simulink model "Batteriemodelle_vergleich"  (R2020a)
settings: Solver=ode15s  StartTime=0.0  StopTime=10.0  MaxStep=1  RelTol=1e-3  AbsTol=1e-3
undefined symbols (not defined in the file or in its folder): c_Mo, J_T, L, M_l, R_a, R_i, R_v, switch_12, switch_48, switch_gen, U_b0
libraries: fl_lib x20, nesl_utility x11, ee_lib x1
settings Model: Creator=ferdi  LastModifiedBy=ferdi
settings SolverCC: AutoScaleAbsTol=off
settings DebuggingCC: SymbolicDimsDataTypeCodeGenerationDiagnostic=none
settings SFSimCC: CustomCodeUndefinedFunction=UseInterfaceOnly
settings SimscapeCC: SimscapeLogType=all  SimscapeLogSimulationStatistics=on  SimscapeLogDataHistory=10000

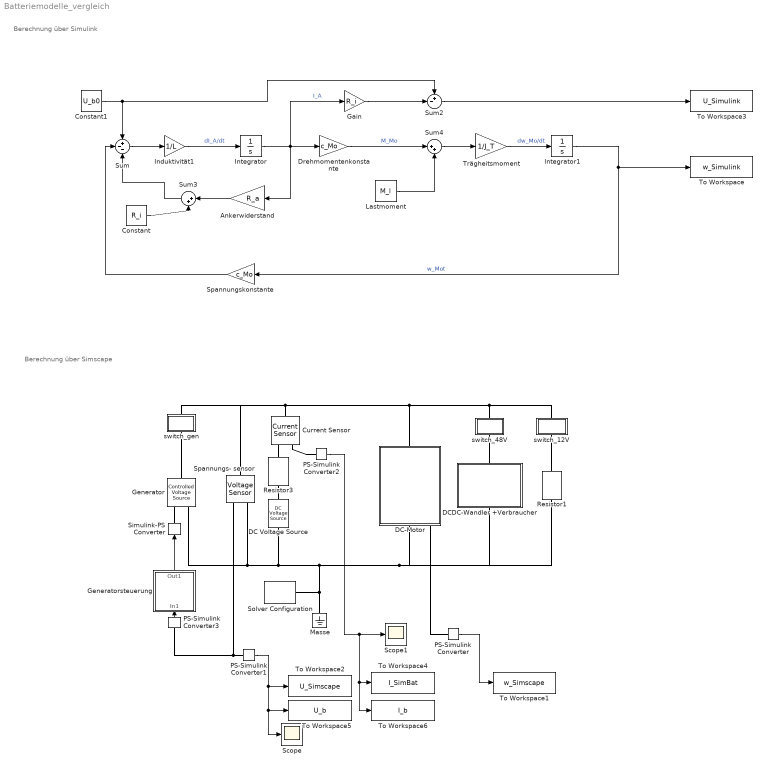
== system Batteriemodelle_vergleich ==
  note: Berechnung über Simscape
  note: Berechnung über Simulink
  Ankerwiderstand : Gain  Gain=R_a
  Constant : Constant  Value=R_i
  Constant1 : Constant  Value=U_b0
  Current Sensor : fl_lib/Electrical/Electrical Sensors/Current Sensor
  DC Voltage Source : fl_lib/Electrical/Electrical Sources/DC Voltage Source  v0=U_b0 V
  DC-Motor : Subsystem
  DCDC-Wandler +Verbraucher : Subsystem
      settings: PortSchema="{\"entries\":[{\"content\":{\"sides\":[{\"content\":{\"connectorIds\":[]},\"type\":\"ConnectorPlacement.EquallySpacedRectSide\",\"uuid\":\"e013d669-d593-4e9e-932c-6ed81a050137\"},{\"content\":{\"connectorIds\":[],\"side\":\"RIGHT\"},\"type\":\"ConnectorPlacement.EquallySpacedRectSide\",\"uuid\":\"a61269dc-61fd-40c3-bd3d-9bfab1dca48c\"},{\"content\":{\"connectorIds\":[\"LConn1\"],\"side\":\"TOP\"},\"type\":\"ConnectorPlacement.EquallySpacedRectSide\",\"uuid\":\"b7f509d6-f5f8-4482-b93c-d65c76c33a27\"},{\"content\":{\"connectorIds\":[\"RConn1\"],\"side\":\"BOTTOM\"},\"type\":\"ConnectorPlacement.EquallySpacedRectSide\",\"uuid\":\"3ea5f8db-940a-44b4-971a-3b24f30d9605\"}]},\"type\":\"ConnectorPlacement.EquallySpacedConnector\",\"uuid\":\"ca129737-90ed-4648-9d71-06bbfa0ff625\"}],\"packageUris\":[\"http://schema.mathworks.com/mf0/Connector/19700101\"],\"version\":\"1.0\"}"
  Drehmomentenkonstante : Gain  Gain=c_Mo
  Gain : Gain  Gain=R_i
  Generator : fl_lib/Electrical/Electrical Sources/Controlled Voltage Source
  Generatorsteuerung : Subsystem
  Induktivität1 : Gain  Gain=1/L
  Integrator : Integrator
  Integrator1 : Integrator
  Lastmoment : Constant  Value=M_l
  Masse : fl_lib/Electrical/Electrical Elements/Electrical Reference
  PS-Simulink Converter{,1..3} (4 alike) : nesl_utility/PS-Simulink Converter  PhysicalDomain=network_engine_domain  SubClassName=ps_output  LeftPortType=input  RightPortType=output  PseudoPeriodic=off  Frequencies=[]  Unit=inherit  AffineConversion=off
      PS-Simulink Converter settings: SourceProductBaseCode=MT,SS
      PS-Simulink Converter1 settings: SourceProductBaseCode=MT,SS
      PS-Simulink Converter2 settings: SourceProductBaseCode=MT,SS
  Resistor1 : fl_lib/Electrical/Electrical Elements/Resistor  R=R_v Ohm  i_specify=off  i_priority=None  i=0 A  i_nominal_specify=off  i_nominal_unit=A  i_nominal_value=1  v_specify=off  v_priority=None  v=0 V  v_nominal_specify=off  v_nominal_unit=V  v_nominal_value=1
  Resistor3 : fl_lib/Electrical/Electrical Elements/Resistor  R=R_i Ohm  i_specify=off  i_priority=None  i=0 A  i_nominal_specify=off  i_nominal_unit=A  i_nominal_value=1  v_specify=off  v_priority=None  v=0 V  v_nominal_specify=off  v_nominal_unit=V  v_nominal_value=1
  Scope : Scope
  Scope1 : Scope
  Simulink-PS Converter : nesl_utility/Simulink-PS Converter  PhysicalDomain=network_engine_domain  SubClassName=ps_input  LeftPortType=input  RightPortType=output  PseudoPeriodic=off  Frequencies=[]  NoiseDistribution=none  NoiseParameters=[]  Unit=1  AffineConversion=off  FilteringAndDerivatives=provide  SimscapeFilterOrder=1  InputFilterTimeConstant=0.001  UdotUserProvided=0
  Solver Configuration : nesl_utility/Solver Configuration  PhysicalDomain=network_engine_domain  SubClassName=solver  LeftPortType=input  RightPortType=generic  Tones=[]  Harmonics=[]  SimulateNoise=off  Profile=off  UseLocalSampling=off  EnableSwitchedLinearOptims=on  FrequencyDomain=off  UseCCode=off  RelTol=0.001  AbsTol=1e-06  MinStep=1e-09  ToWorkspace=off  RevertToSquareIcSolve=off  NumHomotopyIterations=100  PhasorMode=off  PhasorModeNumHarmonics=1  DoDC=off  ResidualTolerance=1e-09  UseLocalSolver=off  LocalSolverChoice=NE_BACKWARD_EULER_ADVANCER  LocalSolverSampleTime=0.001  DoFixedCost=off  MaxNonlinIter=3  MaxModeIter=2  LinearAlgebra=auto  EquationFormulation=NE_TIME_EF  DelaysMemoryBudget=1024  AutomaticFiltering=on  FilteringTimeConstant=0.001  PartitionStorageMethod=AS_NEEDED  PartitionMemoryBudget=1024  PartitionMethod=ROBUST
      settings: SourceProductBaseCode=MT,SS
  Spannungs- sensor : fl_lib/Electrical/Electrical Sensors/Voltage Sensor
  Spannungskonstante : Gain  Gain=c_Mo
  Sum : Sum  Inputs=+--
  Sum2 : Sum  Inputs=+-|
  Sum3 : Sum  Inputs=|++
  Sum4 : Sum  Inputs=|++
  To Workspace : ToWorkspace  VariableName=w_Simulink  SaveFormat=Timeseries  SampleTime=-1
  To Workspace1 : ToWorkspace  VariableName=w_Simscape  SaveFormat=Timeseries  SampleTime=-1
  To Workspace2 : ToWorkspace  VariableName=U_Simscape  SaveFormat=Timeseries  SampleTime=-1
  To Workspace3 : ToWorkspace  VariableName=U_Simulink  SaveFormat=Timeseries  SampleTime=-1
  To Workspace4 : ToWorkspace  VariableName=I_SimBat  SaveFormat=Timeseries  SampleTime=-1
  To Workspace5 : ToWorkspace  VariableName=U_b  SaveFormat=Structure  SampleTime=-1
  To Workspace6 : ToWorkspace  VariableName=I_b  SaveFormat=Structure  SampleTime=-1
  Trägheitsmoment : Gain  Gain=1/J_T
  switch_12V : Subsystem
      settings: PortSchema="{\"entries\":[{\"content\":{\"sides\":[{\"content\":{\"connectorIds\":[]},\"type\":\"ConnectorPlacement.EquallySpacedRectSide\",\"uuid\":\"e657420c-9952-4b84-8f75-dd008fdb8b47\"},{\"content\":{\"connectorIds\":[],\"side\":\"RIGHT\"},\"type\":\"ConnectorPlacement.EquallySpacedRectSide\",\"uuid\":\"9c3f3fea-d300-4de9-8776-01c952d07adf\"},{\"content\":{\"connectorIds\":[\"LConn1\"],\"side\":\"TOP\"},\"type\":\"ConnectorPlacement.EquallySpacedRectSide\",\"uuid\":\"e53ae76e-8c26-476c-b5cb-d6a2a0ed5aec\"},{\"content\":{\"connectorIds\":[\"RConn1\"],\"side\":\"BOTTOM\"},\"type\":\"ConnectorPlacement.EquallySpacedRectSide\",\"uuid\":\"b9b0f109-8250-480b-8b54-fcb23ebda94c\"}]},\"type\":\"ConnectorPlacement.EquallySpacedConnector\",\"uuid\":\"23c687c1-d9e5-4d6e-b79a-d646f86ae07f\"}],\"packageUris\":[\"http://schema.mathworks.com/mf0/Connector/19700101\"],\"version\":\"1.0\"}"
      mask Display: disp('switch')
  switch_48V : Subsystem
      mask Display: disp('switch')
  switch_gen : Subsystem
      mask Display: disp('switch')
  wires:
  PS-Simulink Converter/1 -> To Workspace1/1
  Constant1/1 -> Sum2/1, Sum/1
  Sum3/1 -> Sum/3
  Sum/1 -> Induktivität1/1
  Constant/1 -> Sum3/2
  Ankerwiderstand/1 -> Sum3/1
  Drehmomentenkonstante/1 -> Sum4/1  "M_Mo"
  Integrator1/1 -> To Workspace/1, Spannungskonstante/1  "w_Mot"
  Induktivität1/1 -> Integrator/1  "dI_A/dt"
  Sum4/1 -> Trägheitsmoment/1
  Gain/1 -> Sum2/2
  Trägheitsmoment/1 -> Integrator1/1  "dw_Mo/dt"
  Lastmoment/1 -> Sum4/2
  Spannungskonstante/1 -> Sum/2
  Integrator/1 -> Gain/1, Drehmomentenkonstante/1, Ankerwiderstand/1  "I_A"
  PS-Simulink Converter1/1 -> To Workspace5/1, Scope/1, To Workspace2/1
  PS-Simulink Converter2/1 -> To Workspace6/1, To Workspace4/1, Scope1/1
  Sum2/1 -> To Workspace3/1
  PS-Simulink Converter3/1 -> Generatorsteuerung/1(In1)
  Generatorsteuerung/1(Out1) -> Simulink-PS Converter/1
  connections:
  PS-Simulink Converter1/LConn1 -- Spannungs- sensor/RConn1 -- PS-Simulink Converter3/LConn1
  Resistor3/LConn1 -- DC Voltage Source/LConn1
  PS-Simulink Converter2/LConn1 -- Current Sensor/RConn1
  PS-Simulink Converter/LConn1 -- DC-Motor/RConn3
  Spannungs- sensor/RConn2 -- Generator/RConn2 -- DC Voltage Source/RConn1 -- DC-Motor/RConn2 -- Resistor1/RConn1 -- DCDC-Wandler +Verbraucher/RConn1 -- Solver Configuration/RConn1 -- Masse/LConn1
  switch_48V/LConn1 -- DCDC-Wandler +Verbraucher/LConn1
  switch_12V/RConn1 -- Resistor1/LConn1
  Current Sensor/RConn2 -- Resistor3/RConn1
  switch_12V/LConn1 -- switch_48V/RConn1 -- DC-Motor/LConn1 -- switch_gen/RConn1 -- Spannungs- sensor/LConn1 -- Current Sensor/LConn1
  Simulink-PS Converter/RConn1 -- Generator/RConn1
  Generator/LConn1 -- switch_gen/LConn1

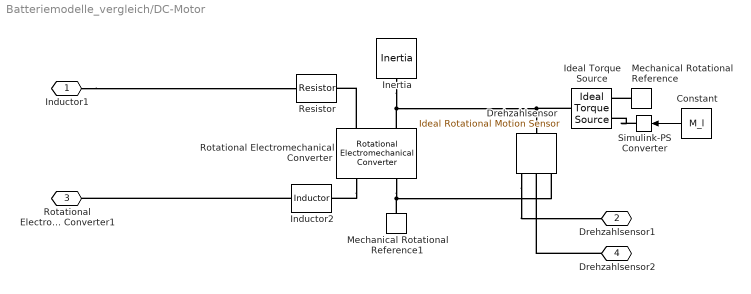
== system Batteriemodelle_vergleich/DC-Motor ==
  Constant : Constant  Value=M_l
  Drehzahlsensor : fl_lib/Mechanical/Mechanical Sensors/Ideal Rotational Motion Sensor  wrap_angle=simscape.enum.onoff.off  offset=0 rad
  Ideal Torque Source : fl_lib/Mechanical/Mechanical Sources/Ideal Torque Source
  Inductor2 : fl_lib/Electrical/Electrical Elements/Inductor  l=L H  r=0 Ohm  g=0 1/Ohm  i_specify=off  i_priority=High  i=3 A  i_nominal_specify=off  i_nominal_unit=A  i_nominal_value=1  v_specify=off  v_priority=None  v=0 V  v_nominal_specify=off  v_nominal_unit=V  v_nominal_value=1  i_L_specify=off  i_L_priority=None  i_L=0 A  i_L_nominal_specify=off  i_L_nominal_unit=A  i_L_nominal_value=1
  Inertia : fl_lib/Mechanical/Rotational Elements/Inertia  inertia=J_T kg*m^2  w_specify=off  w_priority=High  w=0 rad/s  w_nominal_specify=off  w_nominal_unit=rad/s  w_nominal_value=1  t_specify=off  t_priority=None  t=0 N*m  t_nominal_specify=off  t_nominal_unit=N*m  t_nominal_value=1
  Mechanical Rotational Reference : fl_lib/Mechanical/Rotational Elements/Mechanical Rotational Reference
  Mechanical Rotational Reference1 : fl_lib/Mechanical/Rotational Elements/Mechanical Rotational Reference
  Resistor : fl_lib/Electrical/Electrical Elements/Resistor  R=R_a Ohm  i_specify=off  i_priority=High  i=3 A  i_nominal_specify=off  i_nominal_unit=A  i_nominal_value=1  v_specify=off  v_priority=None  v=0 V  v_nominal_specify=off  v_nominal_unit=V  v_nominal_value=1
  Rotational Electromechanical Converter : fl_lib/Electrical/Electrical Elements/Rotational Electromechanical Converter  K=c_Mo V/(rad/s)  i_specify=off  i_priority=None  i=3 A  i_nominal_specify=off  i_nominal_unit=A  i_nominal_value=1  v_specify=off  v_priority=None  v=12 V  v_nominal_specify=off  v_nominal_unit=V  v_nominal_value=1  t_specify=off  t_priority=High  t=-20 N*m  t_nominal_specify=off  t_nominal_unit=N*m  t_nominal_value=1  w_specify=off  w_priority=None  w=0 rad/s  w_nominal_specify=off  w_nominal_unit=rad/s  w_nominal_value=1
  Simulink-PS Converter : nesl_utility/Simulink-PS Converter  PhysicalDomain=network_engine_domain  SubClassName=ps_input  LeftPortType=input  RightPortType=output  PseudoPeriodic=off  Frequencies=[]  NoiseDistribution=none  NoiseParameters=[]  Unit=1  AffineConversion=off  FilteringAndDerivatives=provide  SimscapeFilterOrder=1  InputFilterTimeConstant=0.001  UdotUserProvided=0
  Inductor1 : PMIOPort  Side=Left
  Drehzahlsensor1 : PMIOPort  Port=2  Side=Right
  Rotational Electromechanical Converter1 : PMIOPort  Port=3  Side=Right
  Drehzahlsensor2 : PMIOPort  Port=4  Side=Right
  wires:
  Constant/1 -> Simulink-PS Converter/1
  connections:
  Mechanical Rotational Reference1/LConn1 -- Rotational Electromechanical Converter/RConn2 -- Drehzahlsensor/RConn1
  Inductor1/RConn1 -- Resistor/LConn1
  Inertia/LConn1 -- Rotational Electromechanical Converter/LConn2 -- Ideal Torque Source/LConn1 -- Drehzahlsensor/LConn1
  Rotational Electromechanical Converter/LConn1 -- Resistor/RConn1
  Drehzahlsensor/RConn3 -- Drehzahlsensor1/RConn1
  Drehzahlsensor2/RConn1 -- Drehzahlsensor/RConn2
  Rotational Electromechanical Converter/RConn1 -- Inductor2/RConn1
  Inductor2/LConn1 -- Rotational Electromechanical Converter1/RConn1
  Mechanical Rotational Reference/LConn1 -- Ideal Torque Source/RConn2
  Simulink-PS Converter/RConn1 -- Ideal Torque Source/RConn1

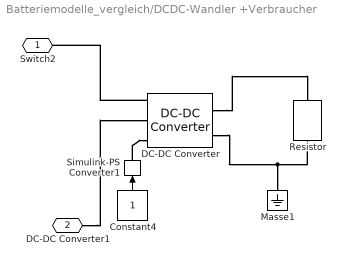
== system Batteriemodelle_vergleich/DCDC-Wandler +Verbraucher ==
  Constant4 : Constant
  DC-DC Converter : ee_lib/Semiconductors & Converters/Converters/DC-DC Converter  Vref_option=ee.enum.converters.voltageref.internal  v_ref=12 V  P_rated=10 W  droop_param=1  droop=0.1 V/A  droop_percent=2  reversible=0  efficiency=80  P_fixed=1 W  model_dynamics=0  tau=0.02 s  v_ini=10 V  G_diode=1e-8 1/Ohm  i1_max=100 A  fault_condition=1  fault_threshold=0.5  thermal_mass=100 J/K  initial_temperature=298.15 K
      settings: SourceProductBaseCode=PS  InternalSimscapePortConfiguration="{\"Bottom\":[],\"Left\":[{\"id\":\"p1\",\"label\":\"1+\",\"type\":\"foundation.electrical.electrical\"},{\"id\":\"n1\",\"label\":\"1-\",\"type\":\"foundation.electrical.electrical\"},{\"id\":\"F\",\"label\":\"F\",\"type\":\"input\"}],\"Right\":[{\"id\":\"p2\",\"label\":\"2+\",\"type\":\"foundation.electrical.electrical\"},{\"id\":\"n2\",\"label\":\"2-\",\"type\":\"foundation.electrical.electrical\"}],\"Top\":[]}"
  Masse1 : fl_lib/Electrical/Electrical Elements/Electrical Reference
  Resistor : fl_lib/Electrical/Electrical Elements/Resistor  R=500 Ohm  i_specify=off  i_priority=None  i=0 A  i_nominal_specify=off  i_nominal_unit=A  i_nominal_value=1  v_specify=off  v_priority=None  v=0 V  v_nominal_specify=off  v_nominal_unit=V  v_nominal_value=1
  Simulink-PS Converter1 : nesl_utility/Simulink-PS Converter  PhysicalDomain=network_engine_domain  SubClassName=ps_input  LeftPortType=input  RightPortType=output  PseudoPeriodic=off  Frequencies=[]  NoiseDistribution=none  NoiseParameters=[]  Unit=1  AffineConversion=off  FilteringAndDerivatives=provide  SimscapeFilterOrder=1  InputFilterTimeConstant=0.001  UdotUserProvided=0
  Switch2 : PMIOPort  Side=Left
  DC-DC Converter1 : PMIOPort  Port=2  Side=Right
  wires:
  Constant4/1 -> Simulink-PS Converter1/1
  connections:
  DC-DC Converter/RConn1 -- Resistor/LConn1
  DC-DC Converter1/RConn1 -- DC-DC Converter/LConn2
  DC-DC Converter/RConn2 -- Masse1/LConn1 -- Resistor/RConn1
  Simulink-PS Converter1/RConn1 -- DC-DC Converter/LConn3
  DC-DC Converter/LConn1 -- Switch2/RConn1

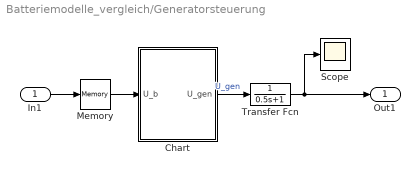
== system Batteriemodelle_vergleich/Generatorsteuerung ==
  In1 : Inport
  Chart : Stateflow chart  TreatAsAtomicUnit=on
  Memory : Memory
  Scope : Scope
  Transfer Fcn : TransferFcn  Denominator=[0.5 1]
  Out1 : Outport
  wires:
  Chart/1(U_gen) -> Transfer Fcn/1  "U_gen"
  Transfer Fcn/1 -> Out1/1, Scope/1
  Memory/1 -> Chart/1(U_b)
  In1/1 -> Memory/1

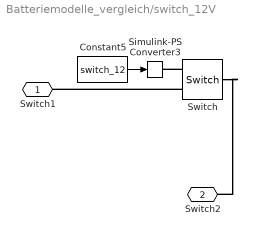
== system Batteriemodelle_vergleich/switch_12V ==
  Constant5 : Constant  Value=switch_12
  Simulink-PS Converter3 : nesl_utility/Simulink-PS Converter  PhysicalDomain=network_engine_domain  SubClassName=ps_input  LeftPortType=input  RightPortType=output  PseudoPeriodic=off  Frequencies=[]  NoiseDistribution=none  NoiseParameters=[]  Unit=1  AffineConversion=off  FilteringAndDerivatives=provide  SimscapeFilterOrder=1  InputFilterTimeConstant=0.001  UdotUserProvided=0
  Switch : fl_lib/Electrical/Electrical Elements/Switch  R_closed=0.01 Ohm  G_open=1e-8 1/Ohm  Threshold=0.5  i_specify=off  i_priority=None  i=0 A  i_nominal_specify=off  i_nominal_unit=A  i_nominal_value=1  v_specify=off  v_priority=None  v=0 V  v_nominal_specify=off  v_nominal_unit=V  v_nominal_value=1
  Switch1 : PMIOPort  Side=Left
  Switch2 : PMIOPort  Port=2  Side=Right
  wires:
  Constant5/1 -> Simulink-PS Converter3/1
  connections:
  Switch/RConn2 -- Switch1/RConn1
  Switch/RConn1 -- Simulink-PS Converter3/RConn1
  Switch/LConn1 -- Switch2/RConn1

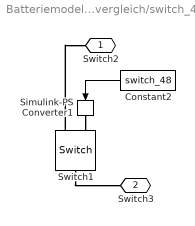
== system Batteriemodelle_vergleich/switch_48V ==
  Constant2 : Constant  Value=switch_48
  Simulink-PS Converter1 : nesl_utility/Simulink-PS Converter  PhysicalDomain=network_engine_domain  SubClassName=ps_input  LeftPortType=input  RightPortType=output  PseudoPeriodic=off  Frequencies=[]  NoiseDistribution=none  NoiseParameters=[]  Unit=1  AffineConversion=off  FilteringAndDerivatives=provide  SimscapeFilterOrder=1  InputFilterTimeConstant=0.001  UdotUserProvided=0
  Switch1 : fl_lib/Electrical/Electrical Elements/Switch  R_closed=0.01 Ohm  G_open=1e-8 1/Ohm  Threshold=0.5  i_specify=off  i_priority=None  i=0 A  i_nominal_specify=off  i_nominal_unit=A  i_nominal_value=1  v_specify=off  v_priority=None  v=0 V  v_nominal_specify=off  v_nominal_unit=V  v_nominal_value=1
  Switch2 : PMIOPort  Side=Right
  Switch3 : PMIOPort  Port=2  Side=Left
  wires:
  Constant2/1 -> Simulink-PS Converter1/1
  connections:
  Switch1/LConn1 -- Switch3/RConn1
  Simulink-PS Converter1/RConn1 -- Switch1/RConn1
  Switch1/RConn2 -- Switch2/RConn1

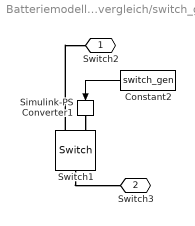
== system Batteriemodelle_vergleich/switch_gen ==
  Constant2 : Constant  Value=switch_gen
  Simulink-PS Converter1 : nesl_utility/Simulink-PS Converter  PhysicalDomain=network_engine_domain  SubClassName=ps_input  LeftPortType=input  RightPortType=output  PseudoPeriodic=off  Frequencies=[]  NoiseDistribution=none  NoiseParameters=[]  Unit=1  AffineConversion=off  FilteringAndDerivatives=provide  SimscapeFilterOrder=1  InputFilterTimeConstant=0.001  UdotUserProvided=0
  Switch1 : fl_lib/Electrical/Electrical Elements/Switch  R_closed=0.01 Ohm  G_open=1e-8 1/Ohm  Threshold=0.5  i_specify=off  i_priority=None  i=0 A  i_nominal_specify=off  i_nominal_unit=A  i_nominal_value=1  v_specify=off  v_priority=None  v=0 V  v_nominal_specify=off  v_nominal_unit=V  v_nominal_value=1
  Switch2 : PMIOPort  Side=Right
  Switch3 : PMIOPort  Port=2  Side=Left
  wires:
  Constant2/1 -> Simulink-PS Converter1/1
  connections:
  Switch1/LConn1 -- Switch3/RConn1
  Simulink-PS Converter1/RConn1 -- Switch1/RConn1
  Switch1/RConn2 -- Switch2/RConn1

== stateflow chart Batteriemodelle_vergleich/Generatorsteuerung/Chart ==
  state system_12V
    state Gen_low
      entry:
      U_gen = 0;
    state Gen_high
      entry:
      U_gen = 12;
    (default) -> Gen_low
    Gen_low -> Gen_high : [U_b <= 11]
    Gen_high -> Gen_low : [U_b > 11.5]
  data: U_gen output; U_b input
